simulink model "ball_on_plate_simulink"  (R2020b)
settings: Solver=VariableStepAuto  StartTime=0.0  StopTime=inf  RelTol=1e-3
model workspace (MAT data in the model file):
  THETA_MAX = 1.57079632679
  THETA_MIN = -1.57079632679
  xcoord = Simulink.Parameter
  xcoord.Value = 0.5
  xcoord.DataType = 'auto'
  xcoord.Dimensions = [1 1]
  ycoord = Simulink.Parameter
  ycoord.Value = 0.5
  ycoord.DataType = 'auto'
  ycoord.Dimensions = [1 1]
settings Model: NumberOfSteps=20  Creator=blake  LastModifiedBy=blake

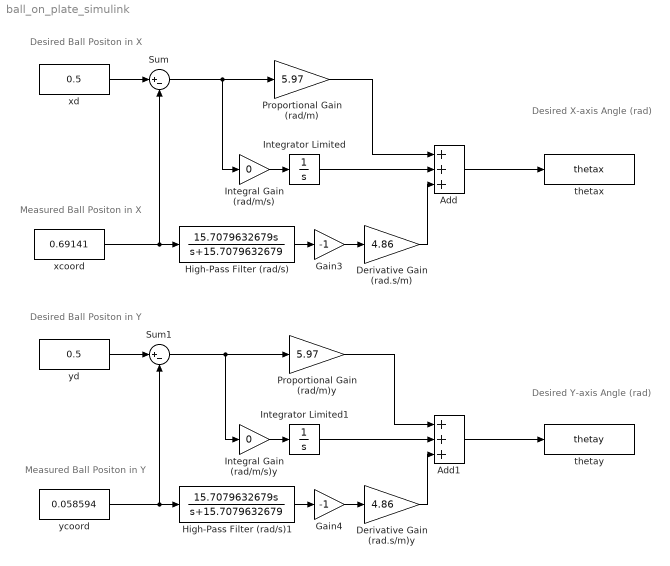
== system ball_on_plate_simulink ==
  note: Measured Ball Positon in X
  note: Desired Ball Positon in X
  note: Measured Ball Positon in Y
  note: Desired Ball Positon in Y
  note: Desired Y-axis Angle (rad)
  note: Desired X-axis Angle (rad)
  Add : Sum  Inputs=+++
  Add1 : Sum  Inputs=+++
  Derivative Gain (rad.s/m) : Gain  Gain=4.86
  Derivative Gain (rad.s/m)y : Gain  Gain=4.86
  Gain3 : Gain  Gain=-1
  Gain4 : Gain  Gain=-1
  High-Pass Filter (rad/s) : TransferFcn  Numerator=[15.7079632679 0]  Denominator=[1 15.7079632679]
  High-Pass Filter (rad/s)1 : TransferFcn  Numerator=[15.7079632679 0]  Denominator=[1 15.7079632679]
  Integral Gain (rad/m/s) : Gain  Gain=0
  Integral Gain (rad/m/s)y : Gain  Gain=0
  Integrator Limited : Integrator  LimitOutput=on  UpperSaturationLimit=20*pi/180  LowerSaturationLimit=-20*pi/180
  Integrator Limited1 : Integrator  LimitOutput=on  UpperSaturationLimit=20*pi/180  LowerSaturationLimit=-20*pi/180
  Proportional Gain (rad/m) : Gain  Gain=5.97
  Proportional Gain (rad/m)y : Gain  Gain=5.97
  Sum : Sum  Inputs=|+-
  Sum1 : Sum  Inputs=|+-
  thetax : ToWorkspace  VariableName=thetax  SaveFormat=Timeseries  SampleTime=-1
  thetay : ToWorkspace  VariableName=thetay  SaveFormat=Timeseries  SampleTime=-1
  xcoord : Constant  Value=0.69141
  xd : Constant  Value=0.5
  ycoord : Constant  Value=0.058594
  yd : Constant  Value=0.5
  wires:
  xd/1 -> Sum/1
  xcoord/1 -> Sum/2, High-Pass Filter (rad/s)/1
  Proportional Gain (rad/m)/1 -> Add/1
  Integrator Limited/1 -> Add/2
  Integral Gain (rad/m/s)/1 -> Integrator Limited/1
  High-Pass Filter (rad/s)/1 -> Gain3/1
  Gain4/1 -> Derivative Gain (rad.s/m)y/1
  High-Pass Filter (rad/s)1/1 -> Gain4/1
  Sum1/1 -> Integral Gain (rad/m/s)y/1, Proportional Gain (rad/m)y/1
  Integral Gain (rad/m/s)y/1 -> Integrator Limited1/1
  Integrator Limited1/1 -> Add1/2
  Derivative Gain (rad.s/m)y/1 -> Add1/3
  Proportional Gain (rad/m)y/1 -> Add1/1
  ycoord/1 -> High-Pass Filter (rad/s)1/1, Sum1/2
  yd/1 -> Sum1/1
  Gain3/1 -> Derivative Gain (rad.s/m)/1
  Add1/1 -> thetay/1
  Add/1 -> thetax/1
  Derivative Gain (rad.s/m)/1 -> Add/3
  Sum/1 -> Integral Gain (rad/m/s)/1, Proportional Gain (rad/m)/1
